simulink model "Mutiphase_inverter"  (Simulink 6.1)
settings: Solver=ode23tb  StartTime=0.0  StopTime=0.1499  MaxStep=5e-5  MinStep=1e-8  RelTol=1e-3  AbsTol=.1
libraries: powerlib x15
settings Model: LastModifiedBy=ThinkPad
settings DebuggingCC: SolverPrmCheckMsg=warning

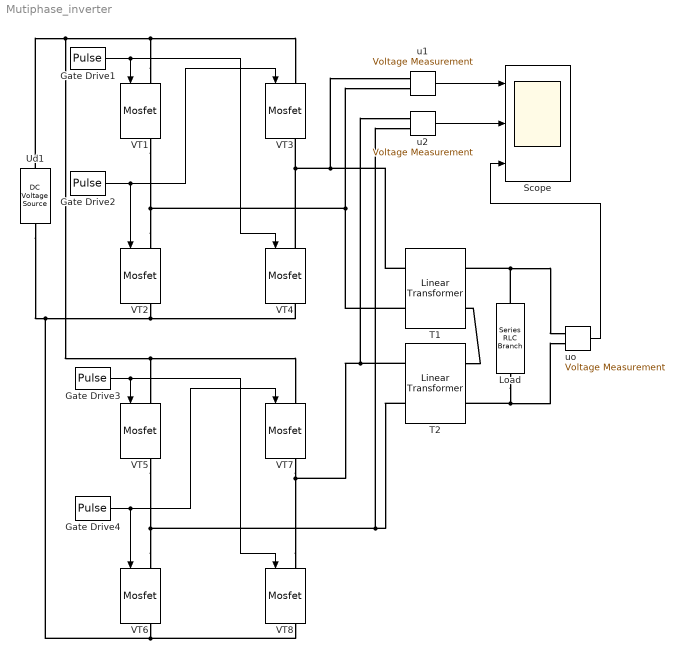
== system Mutiphase_inverter ==
  Gate Drive1 : DiscretePulseGenerator  PulseType=Time based  Period=0.02  PulseWidth=49.5
  Gate Drive2 : DiscretePulseGenerator  PulseType=Time based  Period=0.02  PulseWidth=49.5  PhaseDelay=0.01
  Gate Drive3 : DiscretePulseGenerator  PulseType=Time based  Period=0.02  PulseWidth=49.5  PhaseDelay=0.00333
  Gate Drive4 : DiscretePulseGenerator  PulseType=Time based  Period=0.02  PulseWidth=49.5  PhaseDelay=0.01333
  Load : powerlib/Elements/Series RLC Branch  Orientation=up  PhysicalDomain=powersysdomain  SubClassName=unknown  LeftPortType=p1  RightPortType=p1  LConnTagsString=__new0  RConnTagsString=__new0  Resistance=50  Inductance=0.01  Capacitance=inf  Measurements=Branch voltage and current
  Scope : Scope  NumInputPorts=3
      settings: TickLabels=on  TimeRange=0.05  YMin=-200~-200~-300  YMax=200~200~300  SampleTime=2e-4
  T1 : powerlib/Elements/Linear Transformer  PhysicalDomain=powersysdomain  SubClassName=unknown  LeftPortType=p1  RightPortType=p1  LConnTagsString=a|b  RConnTagsString=A|B  NominalPower=[ 1e4 50 ]  winding1="[ 100 0.002  0.05 ]"  winding2="[ 100  0.002  0.05 ]"  ThreeWindings=off  winding3=[ 60e3 0.005 0.02 ]  RmLm=[ 500 500 ]  Measurements=None
  T2 : powerlib/Elements/Linear Transformer  PhysicalDomain=powersysdomain  SubClassName=unknown  LeftPortType=p1  RightPortType=p1  LConnTagsString=a|b  RConnTagsString=A|B  NominalPower=[ 10000 50 ]  winding1="[ 100  0.002  0.05 ]"  winding2="[ 100  0.002  0.05 ]"  ThreeWindings=off  winding3=[ 60e3 0.005 0.02 ]  RmLm=[ 500 500 ]  Measurements=None
  Ud1 : powerlib/Electrical Sources/DC Voltage Source  Orientation=up  Amplitude=100  Measurements=None
  VT{1..8} (8 alike) : powerlib/Power Electronics/Mosfet  Orientation=down  Ron=0.01  Lon=1e-7  Rd=.01  IC=0  Rs=5  Cs=1e-6  Measurements=on
  u1 : powerlib/Measurements/Voltage Measurement  PhasorSimulation=off  OutputType=Complex  PSBequivalent=0
  u2 : powerlib/Measurements/Voltage Measurement  PhasorSimulation=off  OutputType=Complex  PSBequivalent=0
  uo : powerlib/Measurements/Voltage Measurement  PhasorSimulation=off  OutputType=Complex  PSBequivalent=0
  wires:
  Gate Drive1/1 -> VT4/1, VT1/1
  Gate Drive2/1 -> VT2/1, VT3/1
  u1/1 -> Scope/1
  Gate Drive3/1 -> VT8/1, VT5/1
  Gate Drive4/1 -> VT6/1, VT7/1
  u2/1 -> Scope/2
  uo/1 -> Scope/3
  connections:
  T1/LConn1 -- VT4/LConn1 -- VT3/RConn1 -- u1/LConn1
  T1/LConn2 -- VT1/RConn1 -- VT2/LConn1 -- u1/LConn2
  VT8/RConn1 -- Ud1/LConn1 -- VT4/RConn1 -- VT2/RConn1 -- VT6/RConn1
  Ud1/RConn1 -- VT3/LConn1 -- VT1/LConn1 -- VT7/LConn1 -- VT5/LConn1
  T2/LConn1 -- VT7/RConn1 -- VT8/LConn1 -- u2/LConn1
  T2/LConn2 -- VT5/RConn1 -- VT6/LConn1 -- u2/LConn2
  Load/RConn1 -- T1/RConn1 -- uo/LConn1
  Load/LConn1 -- T2/RConn2 -- uo/LConn2
  T2/RConn1 -- T1/RConn2
